simulink library "Spring_LeftRight_Nonlinear"  (R2025b)
settings: Solver=VariableStepAuto  StartTime=0.0  StopTime=10.0  RelTol=1e-3
libraries: fl_lib x2, Spring_Nonlinear x2
Description:
  | Component of Simscape Vehicle Templates Library
  | 
  | Copyright 2018-2025 The MathWorks, Inc.
settings Model: Creator=smiller  LastModifiedBy=smiller
settings SolverCC: AlgebraicLoopSolver=TrustRegion
settings DataIOCC: ReturnWorkspaceOutputs=off
settings OptimizationCC: ReuseModelBlockBuffer=off
settings DebuggingCC: UnconnectedInputMsg=warning  UnconnectedOutputMsg=warning  UnconnectedLineMsg=warning  ArithmeticOperatorsInVariantConditions=warning
settings ModelReferenceCC: EnableRefExpFcnMdlSchedulingChecks=on
settings SFSimCC: CustomCodeUndefinedFunction=UseInterfaceOnly
settings RTWCC: GPUComputeCapability=3.5  DLArmComputeVersion=19.05

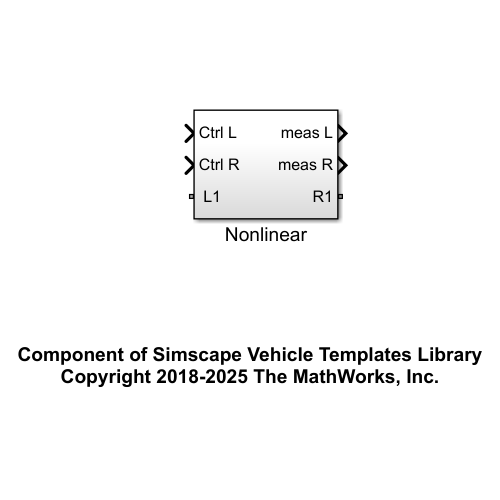
[thumbnail: Simulink's stored preview of the top-level diagram]
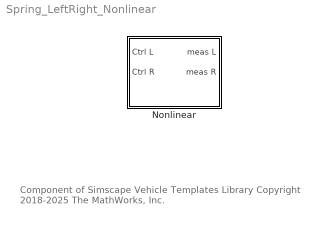
== system Spring_LeftRight_Nonlinear ==
  note: Component of Simscape Vehicle Templates Library
      | Copyright 2018-2025 The MathWorks, Inc.
  Nonlinear : Subsystem  VariantControl=Nonlinear

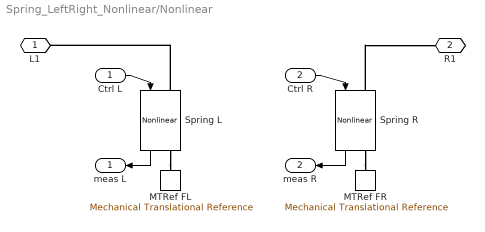
== system Spring_LeftRight_Nonlinear/Nonlinear ==
  Ctrl L : Inport
  Ctrl R : Inport  Port=2
  MTRef FL : fl_lib/Mechanical/Translational Elements/Mechanical Translational Reference
  MTRef FR : fl_lib/Mechanical/Translational Elements/Mechanical Translational Reference
  Spring L : Spring_Nonlinear/Nonlinear  VariantControl=Nonlinear  spr_def0=Spring.xPreload.Value  spr_frc0=Spring.fPreload.Value  deformation_vector=Spring.xSpring.Value  force_vector=Spring.fSpring.Value  spr_hp_top=Spring.sTop.Value  spr_hp_bot=Spring.sBottom.Value
  Spring R : Spring_Nonlinear/Nonlinear  VariantControl=Nonlinear  spr_def0=Spring.xPreload.Value  spr_frc0=Spring.fPreload.Value  deformation_vector=Spring.xSpring.Value  force_vector=Spring.fSpring.Value  spr_hp_top=Spring.sTop.Value  spr_hp_bot=Spring.sBottom.Value
  " L1" : PMIOPort  Side=Left
  R1 : PMIOPort  Port=2  Side=Right
  meas L : Outport  VectorParamsAs1DForOutWhenUnconnected=off
  meas R : Outport  Port=2  VectorParamsAs1DForOutWhenUnconnected=off
  wires:
  Ctrl R/1 -> Spring R/1
  Spring R/1 -> meas R/1
  Spring L/1 -> meas L/1
  Ctrl L/1 -> Spring L/1
  connections:
  Spring R/LConn1 -- R1/RConn1
  Spring L/LConn1 -- " L1"/RConn1
  Spring R/RConn1 -- MTRef FR/LConn1
  Spring L/RConn1 -- MTRef FL/LConn1
